simulink model "LGS_allFaultStuffDeleted"  (R2019b)
settings: Solver=FixedStepDiscrete  StartTime=0.0  StopTime=45.0  FixedStep=0.1  RelTol=1e-3
model workspace (MAT data in the model file):
  fipData : object (value not decoded)
  fipName : object (value not decoded)
  stepSize = 0.1
libraries: commrandsrc3 x16, simulink x3, LibFailureCondition x1
(part 4 of 7)

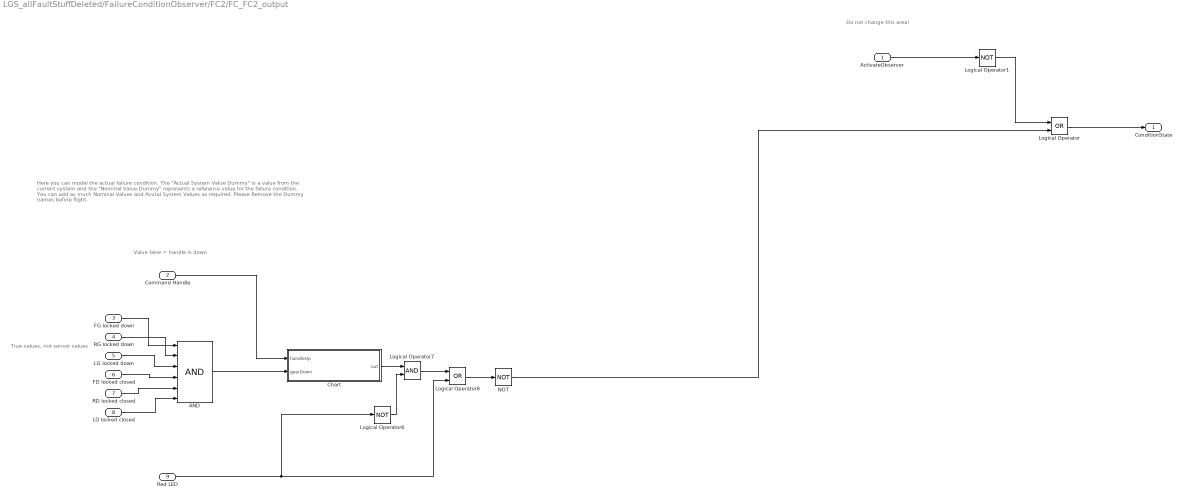
== system LGS_allFaultStuffDeleted/FailureConditionObserver/FC2/FC_FC2_output ==
  note: Here you can model the actual failure condition. The "Actual System Value Dummy" is a value from the current system and the "Nominal Value Dummy"
      | represents a reference value for the failure condition. You can add as much Nominal Values and Acutal System Values as required. Please Remove the
      | Dummy names before flight.
  note: Do not change this area!
  note: True values, not sensor values
  note: Value false = handle is down
  ActivateObserver : Inport
  Command Handle : Inport  Port=2
  FG locked down : Inport  Port=3
  RG locked down : Inport  Port=4
  LG locked down : Inport  Port=5
  FD locked closed : Inport  Port=6
  RD locked closed : Inport  Port=7
  LD locked closed : Inport  Port=8
  Red LED : Inport  Port=9
  AND : Logic  Inputs=6  IconShape=distinctive  AllPortsSameDT=off  OutDataTypeStr=boolean
  Chart : Stateflow chart  TreatAsAtomicUnit=on
  Logical Operator : Logic  Operator=OR  AllPortsSameDT=off  OutDataTypeStr=boolean
  Logical Operator1 : Logic  Operator=NOT  AllPortsSameDT=off  OutDataTypeStr=boolean
  Logical Operator6 : Logic  Operator=NOT  AllPortsSameDT=off  OutDataTypeStr=boolean
  Logical Operator7 : Logic  AllPortsSameDT=off  OutDataTypeStr=boolean
  Logical Operator8 : Logic  Operator=OR  AllPortsSameDT=off  OutDataTypeStr=boolean
  NOT : Logic  Operator=NOT  AllPortsSameDT=off  OutDataTypeStr=boolean
  ConditionState : Outport
  wires:
  ActivateObserver/1 -> Logical Operator1/1
  Logical Operator/1 -> ConditionState/1
  Logical Operator1/1 -> Logical Operator/1
  Logical Operator8/1 -> NOT/1
  Logical Operator7/1 -> Logical Operator8/1
  Logical Operator6/1 -> Logical Operator7/2
  Red LED/1 -> Logical Operator8/2, Logical Operator6/1
  LG locked down/1 -> AND/3
  RD locked closed/1 -> AND/5
  LD locked closed/1 -> AND/6
  FG locked down/1 -> AND/1
  Command Handle/1 -> Chart/1(handleUp)
  Chart/1(out) -> Logical Operator7/1
  RG locked down/1 -> AND/2
  FD locked closed/1 -> AND/4
  AND/1 -> Chart/2(gearDown)
  NOT/1 -> Logical Operator/2

== system LGS_allFaultStuffDeleted/FailureConditionObserver/FC3/ActualSystemCondition ==
  note: This section validates whether the failure condition to be observed will be evaluated. If the
      | last condition evaluates to false, the following conditions will not be evaluated!
      |
      | The last output should be evaluated to a boolean.
  Green LED : Inport
  Orange LED : Inport  Port=2
  Red LED : Inport  Port=3
  AND : Logic  Inputs=3  AllPortsSameDT=off  OutDataTypeStr=boolean
  NOT : Logic  Operator=NOT  AllPortsSameDT=off  OutDataTypeStr=boolean
  NOT1 : Logic  Operator=NOT  AllPortsSameDT=off  OutDataTypeStr=boolean
  "Activate Observer " : Outport
  wires:
  AND/1 -> "Activate Observer "/1
  NOT/1 -> AND/2
  Red LED/1 -> NOT1/1
  Orange LED/1 -> NOT/1
  Green LED/1 -> AND/1
  NOT1/1 -> AND/3

== system LGS_allFaultStuffDeleted/FailureConditionObserver/FC3/FC_FC3_output ==
  note: Here you can model the actual failure condition. The "Actual System Value Dummy" is a value from the current system and the "Nominal Value Dummy"
      | represents a reference value for the failure condition. You can add as much Nominal Values and Acutal System Values as required. Please Remove the
      | Dummy names before flight.
  note: Do not change this area!
  note: True values, not sensor values
  ActivateObserver : Inport
  FG locked down : Inport  Port=2
  RG locked down : Inport  Port=3
  LG locked down : Inport  Port=4
  FD locked closed1 : Inport  Port=5
  RD locked closed1 : Inport  Port=6
  LD locked closed1 : Inport  Port=7
  Logical Operator : Logic  AllPortsSameDT=off  OutDataTypeStr=boolean
  NAND : Logic  Operator=NAND  Inputs=6  IconShape=distinctive  AllPortsSameDT=off  OutDataTypeStr=boolean
  ConditionState : Outport
  wires:
  Logical Operator/1 -> ConditionState/1
  ActivateObserver/1 -> Logical Operator/1
  NAND/1 -> Logical Operator/2
  FG locked down/1 -> NAND/1
  FD locked closed1/1 -> NAND/4
  RD locked closed1/1 -> NAND/5
  RG locked down/1 -> NAND/2
  LG locked down/1 -> NAND/3
  LD locked closed1/1 -> NAND/6

== system LGS_allFaultStuffDeleted/Gears/FG shock absorber/sensor shock absorber ==
  note: [true, false]
  note: [true, false]
  note: [true, false]
  sensor input : Inport  OutDataTypeStr=boolean
  Bus Creator3 : BusCreator  Inputs=3
  FIP1 : Subsystem
  FIP2 : Subsystem
  FIP3 : Subsystem
  sensor output : Outport
  wires:
  FIP2/1(Out1) -> Bus Creator3/2  "signal2"
  FIP1/1(Out1) -> Bus Creator3/1  "signal1"
  FIP3/1(Out1) -> Bus Creator3/3  "signal3"
  sensor input/1 -> FIP3/1(In1), FIP2/1(In1), FIP1/1(In1)
  Bus Creator3/1 -> sensor output/1

== system LGS_allFaultStuffDeleted/Gears/LG shock absorber/sensor shock absorber ==
  note: [true, false]
  note: [true, false]
  sensor input : Inport  OutDataTypeStr=boolean
  Bus Creator3 : BusCreator  Inputs=3
  FIP1 : Subsystem
  FIP2 : Subsystem
  FIP3 : Subsystem
  sensor output : Outport
  wires:
  FIP2/1(Out1) -> Bus Creator3/2  "signal2"
  FIP1/1(Out1) -> Bus Creator3/1  "signal1"
  FIP3/1(Out1) -> Bus Creator3/3  "signal3"
  sensor input/1 -> FIP3/1(In1), FIP2/1(In1), FIP1/1(In1)
  Bus Creator3/1 -> sensor output/1

== system LGS_allFaultStuffDeleted/Gears/RG shock absorber/sensor shock absorber ==
  note: [true, false]
  sensor input : Inport  OutDataTypeStr=boolean
  Bus Creator3 : BusCreator  Inputs=3
  FIP1 : Subsystem
  FIP2 : Subsystem
  FIP3 : Subsystem
  sensor output : Outport
  wires:
  FIP2/1(Out1) -> Bus Creator3/2  "signal2"
  FIP1/1(Out1) -> Bus Creator3/1  "signal1"
  FIP3/1(Out1) -> Bus Creator3/3  "signal3"
  sensor input/1 -> FIP3/1(In1), FIP2/1(In1), FIP1/1(In1)
  Bus Creator3/1 -> sensor output/1

== system LGS_allFaultStuffDeleted/Gears/front gear cylinder/sensor locked extended ==
  note: [true, false]
  note: [true, false]
  note: [true, false]
  sensor input : Inport  OutDataTypeStr=boolean
  Bus Creator3 : BusCreator  Inputs=3
  FIP1 : Subsystem
  FIP2 : Subsystem
  FIP3 : Subsystem
  sensor output : Outport
  wires:
  FIP2/1(Out1) -> Bus Creator3/2  "signal2"
  FIP1/1(Out1) -> Bus Creator3/1  "signal1"
  FIP3/1(Out1) -> Bus Creator3/3  "signal3"
  sensor input/1 -> FIP3/1(In1), FIP2/1(In1), FIP1/1(In1)
  Bus Creator3/1 -> sensor output/1

== system LGS_allFaultStuffDeleted/Gears/front gear cylinder/sensor locked retracted ==
  note: [true, false]
  note: [true, false]
  note: [true, false]
  sensor input : Inport  OutDataTypeStr=boolean
  Bus Creator3 : BusCreator  Inputs=3
  FIP1 : Subsystem
  FIP2 : Subsystem
  FIP3 : Subsystem
  sensor output : Outport
  wires:
  FIP2/1(Out1) -> Bus Creator3/2  "signal2"
  FIP1/1(Out1) -> Bus Creator3/1  "signal1"
  FIP3/1(Out1) -> Bus Creator3/3  "signal3"
  sensor input/1 -> FIP3/1(In1), FIP2/1(In1), FIP1/1(In1)
  Bus Creator3/1 -> sensor output/1

== system LGS_allFaultStuffDeleted/Gears/left gear cylinder/sensor locked extended ==
  note: [true, false]
  note: [true, false]
  note: [true, false]
  sensor input : Inport  OutDataTypeStr=boolean
  Bus Creator3 : BusCreator  Inputs=3
  FIP1 : Subsystem
  FIP2 : Subsystem
  FIP3 : Subsystem
  sensor output : Outport
  wires:
  FIP2/1(Out1) -> Bus Creator3/2  "signal2"
  FIP1/1(Out1) -> Bus Creator3/1  "signal1"
  FIP3/1(Out1) -> Bus Creator3/3  "signal3"
  sensor input/1 -> FIP1/1(In1), FIP2/1(In1), FIP3/1(In1)
  Bus Creator3/1 -> sensor output/1

== system LGS_allFaultStuffDeleted/Gears/left gear cylinder/sensor locked retracted ==
  note: [true, false]
  note: [true, false]
  note: [true, false]
  sensor input : Inport  OutDataTypeStr=boolean
  Bus Creator3 : BusCreator  Inputs=3
  FIP1 : Subsystem
  FIP2 : Subsystem
  FIP3 : Subsystem
  sensor output : Outport
  wires:
  FIP2/1(Out1) -> Bus Creator3/2  "signal2"
  FIP1/1(Out1) -> Bus Creator3/1  "signal1"
  FIP3/1(Out1) -> Bus Creator3/3  "signal3"
  sensor input/1 -> FIP3/1(In1), FIP2/1(In1), FIP1/1(In1)
  Bus Creator3/1 -> sensor output/1

== system LGS_allFaultStuffDeleted/Gears/right gear cylinder/sensor locked extended ==
  note: [true, false]
  note: [true, false]
  note: [true, false]
  sensor input : Inport  OutDataTypeStr=boolean
  Bus Creator3 : BusCreator  Inputs=3
  FIP1 : Subsystem
  FIP2 : Subsystem
  FIP3 : Subsystem
  sensor output : Outport
  wires:
  FIP2/1(Out1) -> Bus Creator3/2  "signal2"
  FIP1/1(Out1) -> Bus Creator3/1  "signal1"
  FIP3/1(Out1) -> Bus Creator3/3  "signal3"
  sensor input/1 -> FIP2/1(In1), FIP3/1(In1), FIP1/1(In1)
  Bus Creator3/1 -> sensor output/1

== system LGS_allFaultStuffDeleted/Gears/right gear cylinder/sensor locked retracted ==
  note: [true, false]
  note: [true, false]
  note: [true, false]
  sensor input : Inport  OutDataTypeStr=boolean
  Bus Creator3 : BusCreator  Inputs=3
  FIP1 : Subsystem
  FIP2 : Subsystem
  FIP3 : Subsystem
  sensor output : Outport
  wires:
  FIP2/1(Out1) -> Bus Creator3/2  "signal2"
  FIP1/1(Out1) -> Bus Creator3/1  "signal1"
  FIP3/1(Out1) -> Bus Creator3/3  "signal3"
  sensor input/1 -> FIP3/1(In1), FIP2/1(In1), FIP1/1(In1)
  Bus Creator3/1 -> sensor output/1

== system LGS_allFaultStuffDeleted/Doors/front door zylinder/sensor locked closed/FIP1 ==
  In1 : Inport
  Out1 : Outport
  wires:
  In1/1 -> Out1/1

== system LGS_allFaultStuffDeleted/Doors/front door zylinder/sensor locked closed/FIP2 ==
  In1 : Inport
  Out1 : Outport
  wires:
  In1/1 -> Out1/1

== system LGS_allFaultStuffDeleted/Doors/front door zylinder/sensor locked closed/FIP3 ==
  In1 : Inport
  Out1 : Outport
  wires:
  In1/1 -> Out1/1

== system LGS_allFaultStuffDeleted/Doors/front door zylinder/sensor open/FIP1 ==
  In1 : Inport
  Out1 : Outport
  wires:
  In1/1 -> Out1/1

== system LGS_allFaultStuffDeleted/Doors/front door zylinder/sensor open/FIP2 ==
  In1 : Inport
  Out1 : Outport
  wires:
  In1/1 -> Out1/1

== system LGS_allFaultStuffDeleted/Doors/front door zylinder/sensor open/FIP3 ==
  In1 : Inport
  Out1 : Outport
  wires:
  In1/1 -> Out1/1

== system LGS_allFaultStuffDeleted/Doors/left door zylinder/sensor locked closed/FIP1 ==
  In1 : Inport
  Out1 : Outport
  wires:
  In1/1 -> Out1/1

== system LGS_allFaultStuffDeleted/Doors/left door zylinder/sensor locked closed/FIP2 ==
  In1 : Inport
  Out1 : Outport
  wires:
  In1/1 -> Out1/1

== system LGS_allFaultStuffDeleted/Doors/left door zylinder/sensor locked closed/FIP3 ==
  In1 : Inport
  Out1 : Outport
  wires:
  In1/1 -> Out1/1

== system LGS_allFaultStuffDeleted/Doors/left door zylinder/sensor open/FIP1 ==
  In1 : Inport
  Out1 : Outport
  wires:
  In1/1 -> Out1/1

== system LGS_allFaultStuffDeleted/Doors/left door zylinder/sensor open/FIP2 ==
  In1 : Inport
  Out1 : Outport
  wires:
  In1/1 -> Out1/1

== system LGS_allFaultStuffDeleted/Doors/left door zylinder/sensor open/FIP3 ==
  In1 : Inport
  Out1 : Outport
  wires:
  In1/1 -> Out1/1

== system LGS_allFaultStuffDeleted/Doors/right door zylinder/sensor locked closed/FIP1 ==
  In1 : Inport
  Out1 : Outport
  wires:
  In1/1 -> Out1/1

== system LGS_allFaultStuffDeleted/Doors/right door zylinder/sensor locked closed/FIP2 ==
  In1 : Inport
  Out1 : Outport
  wires:
  In1/1 -> Out1/1

== system LGS_allFaultStuffDeleted/Doors/right door zylinder/sensor locked closed/FIP3 ==
  In1 : Inport
  Out1 : Outport
  wires:
  In1/1 -> Out1/1

== system LGS_allFaultStuffDeleted/Doors/right door zylinder/sensor open/FIP1 ==
  In1 : Inport
  Out1 : Outport
  wires:
  In1/1 -> Out1/1

== system LGS_allFaultStuffDeleted/Doors/right door zylinder/sensor open/FIP2 ==
  In1 : Inport
  Out1 : Outport
  wires:
  In1/1 -> Out1/1

== system LGS_allFaultStuffDeleted/Doors/right door zylinder/sensor open/FIP3 ==
  In1 : Inport
  Out1 : Outport
  wires:
  In1/1 -> Out1/1

== system LGS_allFaultStuffDeleted/Gears/FG shock absorber/sensor shock absorber/FIP1 ==
  In1 : Inport
  Out1 : Outport
  wires:
  In1/1 -> Out1/1

== system LGS_allFaultStuffDeleted/Gears/FG shock absorber/sensor shock absorber/FIP2 ==
  In1 : Inport
  Out1 : Outport
  wires:
  In1/1 -> Out1/1

== system LGS_allFaultStuffDeleted/Gears/FG shock absorber/sensor shock absorber/FIP3 ==
  In1 : Inport
  Out1 : Outport
  wires:
  In1/1 -> Out1/1

== system LGS_allFaultStuffDeleted/Gears/LG shock absorber/sensor shock absorber/FIP1 ==
  In1 : Inport
  Out1 : Outport
  wires:
  In1/1 -> Out1/1

== system LGS_allFaultStuffDeleted/Gears/LG shock absorber/sensor shock absorber/FIP2 ==
  In1 : Inport
  Out1 : Outport
  wires:
  In1/1 -> Out1/1

== system LGS_allFaultStuffDeleted/Gears/LG shock absorber/sensor shock absorber/FIP3 ==
  In1 : Inport
  Out1 : Outport
  wires:
  In1/1 -> Out1/1

== system LGS_allFaultStuffDeleted/Gears/RG shock absorber/sensor shock absorber/FIP1 ==
  In1 : Inport
  Out1 : Outport
  wires:
  In1/1 -> Out1/1

== system LGS_allFaultStuffDeleted/Gears/RG shock absorber/sensor shock absorber/FIP2 ==
  In1 : Inport
  Out1 : Outport
  wires:
  In1/1 -> Out1/1

== system LGS_allFaultStuffDeleted/Gears/RG shock absorber/sensor shock absorber/FIP3 ==
  In1 : Inport
  Out1 : Outport
  wires:
  In1/1 -> Out1/1

== system LGS_allFaultStuffDeleted/Gears/front gear cylinder/sensor locked extended/FIP1 ==
  In1 : Inport
  Out1 : Outport
  wires:
  In1/1 -> Out1/1

== system LGS_allFaultStuffDeleted/Gears/front gear cylinder/sensor locked extended/FIP2 ==
  In1 : Inport
  Out1 : Outport
  wires:
  In1/1 -> Out1/1

== system LGS_allFaultStuffDeleted/Gears/front gear cylinder/sensor locked extended/FIP3 ==
  In1 : Inport
  Out1 : Outport
  wires:
  In1/1 -> Out1/1

== system LGS_allFaultStuffDeleted/Gears/front gear cylinder/sensor locked retracted/FIP1 ==
  In1 : Inport
  Out1 : Outport
  wires:
  In1/1 -> Out1/1

== system LGS_allFaultStuffDeleted/Gears/front gear cylinder/sensor locked retracted/FIP2 ==
  In1 : Inport
  Out1 : Outport
  wires:
  In1/1 -> Out1/1

== system LGS_allFaultStuffDeleted/Gears/front gear cylinder/sensor locked retracted/FIP3 ==
  In1 : Inport
  Out1 : Outport
  wires:
  In1/1 -> Out1/1

== system LGS_allFaultStuffDeleted/Gears/left gear cylinder/sensor locked extended/FIP1 ==
  In1 : Inport
  Out1 : Outport
  wires:
  In1/1 -> Out1/1

== system LGS_allFaultStuffDeleted/Gears/left gear cylinder/sensor locked extended/FIP2 ==
  In1 : Inport
  Out1 : Outport
  wires:
  In1/1 -> Out1/1

== system LGS_allFaultStuffDeleted/Gears/left gear cylinder/sensor locked extended/FIP3 ==
  In1 : Inport
  Out1 : Outport
  wires:
  In1/1 -> Out1/1

== system LGS_allFaultStuffDeleted/Gears/left gear cylinder/sensor locked retracted/FIP1 ==
  In1 : Inport
  Out1 : Outport
  wires:
  In1/1 -> Out1/1

== system LGS_allFaultStuffDeleted/Gears/left gear cylinder/sensor locked retracted/FIP2 ==
  In1 : Inport
  Out1 : Outport
  wires:
  In1/1 -> Out1/1

== system LGS_allFaultStuffDeleted/Gears/left gear cylinder/sensor locked retracted/FIP3 ==
  In1 : Inport
  Out1 : Outport
  wires:
  In1/1 -> Out1/1

== system LGS_allFaultStuffDeleted/Gears/right gear cylinder/sensor locked extended/FIP1 ==
  In1 : Inport
  Out1 : Outport
  wires:
  In1/1 -> Out1/1

== system LGS_allFaultStuffDeleted/Gears/right gear cylinder/sensor locked extended/FIP2 ==
  In1 : Inport
  Out1 : Outport
  wires:
  In1/1 -> Out1/1

== system LGS_allFaultStuffDeleted/Gears/right gear cylinder/sensor locked extended/FIP3 ==
  In1 : Inport
  Out1 : Outport
  wires:
  In1/1 -> Out1/1

== system LGS_allFaultStuffDeleted/Gears/right gear cylinder/sensor locked retracted/FIP1 ==
  In1 : Inport
  Out1 : Outport
  wires:
  In1/1 -> Out1/1

== system LGS_allFaultStuffDeleted/Gears/right gear cylinder/sensor locked retracted/FIP2 ==
  In1 : Inport
  Out1 : Outport
  wires:
  In1/1 -> Out1/1

== system LGS_allFaultStuffDeleted/Gears/right gear cylinder/sensor locked retracted/FIP3 ==
  In1 : Inport
  Out1 : Outport
  wires:
  In1/1 -> Out1/1

== stateflow chart LGS_allFaultStuffDeleted/Analogical switch and general electro-valve and pressure sensor/Analogical switch/analog Switch ==
  state state_analogSwitchOpenFail
    en: analogSwitchState = false;
  state state_analogSwitchOpen
    en: analogSwitchState = false;
    en: time = int8(1);
    du: time = time - 1;
  state state_analogSwitchOpened
    en: analogSwitchState = false;
  state state_analogSwitchClose
    en: analogSwitchState = false;
  state state_analogSwitchClosed
    en: analogSwitchState = true;
    en: time = int8(19);
    du: time = time - 1;
  state state_analogSwitchClosedFail
    en: analogSwitchState = true;
  state_analogSwitchOpen -> state_analogSwitchOpenFail [order 3] : [fail]
  (default) -> state_analogSwitchOpened
  state_analogSwitchOpen -> state_analogSwitchOpened [order 1] : [((time==0) && ~handleStateChanged) && ~fail]
  state_analogSwitchOpen -> state_analogSwitchClose [order 2] : [handleStateChanged && ~fail]
  state_analogSwitchOpened -> state_analogSwitchClose : [handleStateChanged && ~fail]
  state_analogSwitchClosed -> state_analogSwitchOpen [order 1] : [((time==0) && ~handleStateChanged) && ~fail]
  state_analogSwitchClose -> state_analogSwitchClosed
  state_analogSwitchClosed -> state_analogSwitchClosed [order 2] : [handleStateChanged && ~fail]
  state_analogSwitchClosed -> state_analogSwitchClosedFail [order 3] : [fail]
  data: handleStateChanged input boolean; analogSwitchState output boolean [0..1]; time local int8 [0..19]; fail input

== stateflow chart LGS_allFaultStuffDeleted/Digital Part/Computing module1/AnalogicalSwitchMonitoring ==
  state SwitchOpened
    entry: time = int8(21);
    during: time = time -1;
  note: If the analogical switch is seen closed 1.5 second after a time interval of 20
      | seconds during which the handle position has not changed, then the switch
      | is considered as invalid.
  state Idle
    entry: anomaly = false;
  state HandleMoved
  state CounterOrder
  note: If the analogical switch is seen open 1 second after the handle position has
      | changed, then the switch is considered as invalid.
  state Anomaly
    entry: anomaly = true;
  (default) -> Idle
  SwitchOpened -> Idle [order 2] : [((time == 0) && (~SwitchSignal))]
  HandleMoved -> SwitchOpened [order 2] : [((SwitchSignal) && (~HandleMoved))]
  SwitchOpened -> CounterOrder [order 3] : [(HandleMoved)]
  SwitchOpened -> Anomaly [order 1] : [((time == 0) && (SwitchSignal))]
  Idle -> HandleMoved : [(HandleMoved)]
  HandleMoved -> CounterOrder [order 3] : [(HandleMoved)]
  CounterOrder -> HandleMoved
  HandleMoved -> Anomaly [order 1] : [((~SwitchSignal) && (~HandleMoved))]
  data: HandleMoved input boolean; time local int8 [0..21]; SwitchSignal input boolean; anomaly output boolean

== stateflow chart LGS_allFaultStuffDeleted/Analogical switch and general electro-valve and pressure sensor/General EV/general EV ==
  state state_generalEVOpened
    en: generalEVPresure_out = false;
  state state_genralEVClose
    en: generalEVPresure_out = false;
  state state_generalEVClosed
    en: generalEVPresure_out = true;
  (default) -> state_generalEVOpened
  state_generalEVClosed -> state_generalEVOpened : [((~signal_in) || (~generalEVPresure_in)) && ~fail]
  state_generalEVOpened -> state_genralEVClose : [(signal_in && generalEVPresure_in && ~fail)]
  state_genralEVClose -> state_generalEVOpened [order 2] : [((~signal_in) || (~generalEVPresure_in)) && ~fail]
  state_genralEVClose -> state_generalEVClosed [order 1] : [(signal_in && generalEVPresure_in && ~fail)]
  data: generalEVPresure_in input boolean; signal_in input boolean; generalEVPresure_out output boolean [0..1]; fail input

== stateflow chart LGS_allFaultStuffDeleted/Digital Part/Computing module1/DoorMotionMonitoring ==
  state Idle
    entry: anomaly = false;
  state CloseDoors
    entry: time = int8(6);
    during: time = time -1;
  note: if the control software does not see the value door closed[x] = true for all
      | x ∈ {front, left, right} 7 seconds after stimulation of the closure electro-valve,
      | then the doors are considered as blocked and an anomaly is detected.
  state Succeeded
  state OpenDoors
    entry: time = int8(6);
    during: time = time - 1;
  note: if the control software does not see the value door open[x] = false for all x ∈ {front, left, right} 7 seconds after stimulation of the closure electro-valve, then the doors are considered as blocked and an anomaly is detected.
  state CounterOrder
  note: if the control software does not see the value door open[x] = true for all
      | x ∈ {front, left, right} 7 seconds after stimulation of the opening electrovalve,
      | then the doors are considered as blocked and an anomaly is detected.
  state DoorsBlocked
    entry: anomaly = true;
  note: if the control software does not see the value door closed[x] = false for all
      | x ∈ {front, left, right} 7 seconds after stimulation of the opening electro-valve,
      | then the doors are considered as blocked and an anomaly is detected.
  (default) -> Idle
  CloseDoors -> DoorsBlocked [order 2] : [((time == 0) && (~AllDoorsClosed))]
  Idle -> CloseDoors [order 2] : [((CloseDoorValve) && (~AllDoorsClosed))]
  CloseDoors -> DoorsBlocked [order 3] : [((time == 0) && (AllDoorsOpen))]
  Succeeded -> Idle
  CloseDoors -> Succeeded [order 1] : [(((time == 0) && (AllDoorsClosed)) && (~AllDoorsOpen))]
  CounterOrder -> CloseDoors [order 2] : [(CloseDoorValve)]
  CloseDoors -> CounterOrder [order 4] : [(~CloseDoorValve)]
  Idle -> OpenDoors [order 1] : [((OpenDoorValve) && (~AllDoorsOpen))]
  OpenDoors -> Succeeded [order 2] : [(((time == 0) && (~AllDoorsClosed)) && (AllDoorsOpen))]
  CounterOrder -> OpenDoors [order 1] : [(OpenDoorValve)]
  OpenDoors -> CounterOrder [order 4] : [(~OpenDoorValve)]
  OpenDoors -> DoorsBlocked [order 1] : [((time == 0) && (AllDoorsClosed))]
  OpenDoors -> DoorsBlocked [order 3] : [((time == 0) && (~AllDoorsOpen))]
  data: OpenDoorValve input boolean; time local int8 [0..6]; CloseDoorValve input boolean; anomaly output boolean; AllDoorsClosed input boolean; AllDoorsOpen input boolean

== stateflow chart LGS_allFaultStuffDeleted/Digital Part/Computing module1/GearMotionMonitoring ==
  state ContinueExtending
    entry: time = int8(2);
    during: time = time -1;
  note: if the control software does not see the value gear extended[x] = true for all x ∈ {front, left, right} 10 seconds after stimulation of the extension electrovalve, then the gears are considered as blocked and an anomaly is detected.
  state Idle
    entry: anomaly = false;
  state ExtendGears
    entry: time = int8(6);
    during: time = time -1;
  state RetractGears
    entry: time = int8(6);
    during: time = time - 1;
  state ContinueRetracting
    entry: time = int8(2);
    during: time = time -1;
  state Succeeded
  note: if the control software does not see the value gear retracted[x] = false for all x ∈ {front, left, right} 7 seconds after stimulation of the extension electrovalve, then the gears are considered as blocked and an anomaly is detected.
  state GearsBlocked
    entry: anomaly = true;
  state CounterOrder
  note: if the control software does not see the value gear retracted[x] = true for all x ∈ {front, left, right} 10 seconds after stimulation of the retraction electrovalve, then the gears are considered as blocked and an anomaly is detected.
  note: if the control software does not see the value gear extended[x] = false for all
      | x ∈ {front, left, right} 7 seconds after stimulation of the retraction electrovalve,
      | then the gears are considered as blocked and an anomaly is detected.
  (default) -> Idle
  ExtendGears -> ContinueExtending [order 1] : [((time == 0) && (~AllGearsRetracted))]
  Idle -> ExtendGears [order 2] : [(ExtensionValve)]
  ExtendGears -> GearsBlocked [order 2] : [((time == 0) && (AllGearsRetracted))]
  Succeeded -> Idle
  ExtendGears -> CounterOrder [order 3] : [(~ExtensionValve)]
  ContinueExtending -> GearsBlocked [order 2] : [((time == 0) && (~AllGearsExtended))]
  CounterOrder -> ExtendGears [order 2] : [(ExtensionValve)]
  Idle -> RetractGears [order 1] : [(RetractionValve)]
  ContinueExtending -> CounterOrder [order 3] : [(~ExtensionValve)]
  ContinueExtending -> Succeeded [order 1] : [((time == 0) && (AllGearsExtended))]
  RetractGears -> ContinueRetracting [order 2] : [((time == 0) && (~AllGearsExtended))]
  ContinueRetracting -> Succeeded [order 1] : [((time == 0) && (AllGearsRetracted))]
  CounterOrder -> RetractGears [order 1] : [(RetractionValve)]
  ContinueRetracting -> GearsBlocked [order 2] : [((time == 0) && (~AllGearsRetracted))]
  RetractGears -> GearsBlocked [order 1] : [((time == 0) && (AllGearsExtended))]
  RetractGears -> CounterOrder [order 3] : [(~RetractionValve)]
  ContinueRetracting -> CounterOrder [order 3] : [(~RetractionValve)]
  data: time local int8 [0..6]; anomaly output boolean; AllGearsExtended input boolean; AllGearsRetracted input boolean; ExtensionValve input boolean; RetractionValve input boolean

== stateflow chart LGS_allFaultStuffDeleted/Digital Part/Computing module1/GenericMonitoring/GenericMonitoring2 ==
  state SensorValid
    entry: anomaly = false;
  state Channel1Invalid
  state SensorInvalid
    entry: anomaly = true;
  note: If at t the three channels are considered as valid and are equal, then the
      | value considered by the control software is this common value.
  state Channel2Invalid
  note: If a channel has been eliminated previously, and if at t the two remaining
      | channels are not equal, then the sensor is definitely considered as invalid.
  state Channel3Invalid
  note: If at t one channel is different from the two others for the first time (i.e.,
      | the three channels were considered as valid up to t), then this channel is
      | considered as invalid and is definitely eliminated. Only the two remaining
      | channels are considered in the future. At time t, the value considered by the
      | control software is the common value of the two remaining channels.
  (default) -> SensorValid
  SensorValid -> Channel1Invalid [order 1] : [(((Channel3&&Channel2) || ((~Channel3)&&(~Channel2))) && ((Channel1 && (~Channel2)) || ((~Channel1) && Channel2)))]
  Channel1Invalid -> SensorInvalid : [((Channel2 && (~Channel3)) || ((~Channel2) && Channel3))]
  SensorValid -> Channel2Invalid [order 2] : [(((Channel1&&Channel3) || ((~Channel1)&&(~Channel3))) && ((Channel1 && (~Channel2)) || ((~Channel1) && Channel2)))]
  SensorValid -> Channel3Invalid [order 3] : [(((Channel1&&Channel2) || ((~Channel1)&&(~Channel2))) && ((Channel1 && (~Channel3)) || ((~Channel1) && Channel3)))]
  Channel2Invalid -> SensorInvalid : [((Channel1 && (~Channel3)) || ((~Channel1) && Channel3))]
  Channel3Invalid -> SensorInvalid : [((Channel2 && (~Channel1)) || ((~Channel2) && Channel1))]
  data: Channel1 input boolean; Channel2 input boolean; Channel3 input boolean; anomaly output boolean

== stateflow chart LGS_allFaultStuffDeleted/Digital Part/Computing module1/GenericMonitoring1/GenericMonitoring2 ==
  state SensorValid
    entry: anomaly = false;
  state Channel1Invalid
  state SensorInvalid
    entry: anomaly = true;
  note: If at t the three channels are considered as valid and are equal, then the
      | value considered by the control software is this common value.
  state Channel2Invalid
  note: If a channel has been eliminated previously, and if at t the two remaining
      | channels are not equal, then the sensor is definitely considered as invalid.
  state Channel3Invalid
  note: If at t one channel is different from the two others for the first time (i.e.,
      | the three channels were considered as valid up to t), then this channel is
      | considered as invalid and is definitely eliminated. Only the two remaining
      | channels are considered in the future. At time t, the value considered by the
      | control software is the common value of the two remaining channels.
  (default) -> SensorValid
  SensorValid -> Channel1Invalid [order 1] : [(((Channel3&&Channel2) || ((~Channel3)&&(~Channel2))) && ((Channel1 && (~Channel2)) || ((~Channel1) && Channel2)))]
  Channel1Invalid -> SensorInvalid : [((Channel2 && (~Channel3)) || ((~Channel2) && Channel3))]
  SensorValid -> Channel2Invalid [order 2] : [(((Channel1&&Channel3) || ((~Channel1)&&(~Channel3))) && ((Channel1 && (~Channel2)) || ((~Channel1) && Channel2)))]
  SensorValid -> Channel3Invalid [order 3] : [(((Channel1&&Channel2) || ((~Channel1)&&(~Channel2))) && ((Channel1 && (~Channel3)) || ((~Channel1) && Channel3)))]
  Channel2Invalid -> SensorInvalid : [((Channel1 && (~Channel3)) || ((~Channel1) && Channel3))]
  Channel3Invalid -> SensorInvalid : [((Channel2 && (~Channel1)) || ((~Channel2) && Channel1))]
  data: Channel1 input boolean; Channel2 input boolean; Channel3 input boolean; anomaly output boolean

== stateflow chart LGS_allFaultStuffDeleted/Digital Part/Computing module1/GenericMonitoring10/GenericMonitoring2 ==
  state SensorValid
    entry: anomaly = false;
  state Channel1Invalid
  state SensorInvalid
    entry: anomaly = true;
  note: If at t the three channels are considered as valid and are equal, then the
      | value considered by the control software is this common value.
  state Channel2Invalid
  note: If a channel has been eliminated previously, and if at t the two remaining
      | channels are not equal, then the sensor is definitely considered as invalid.
  state Channel3Invalid
  note: If at t one channel is different from the two others for the first time (i.e.,
      | the three channels were considered as valid up to t), then this channel is
      | considered as invalid and is definitely eliminated. Only the two remaining
      | channels are considered in the future. At time t, the value considered by the
      | control software is the common value of the two remaining channels.
  (default) -> SensorValid
  SensorValid -> Channel1Invalid [order 1] : [(((Channel3&&Channel2) || ((~Channel3)&&(~Channel2))) && ((Channel1 && (~Channel2)) || ((~Channel1) && Channel2)))]
  Channel1Invalid -> SensorInvalid : [((Channel2 && (~Channel3)) || ((~Channel2) && Channel3))]
  SensorValid -> Channel2Invalid [order 2] : [(((Channel1&&Channel3) || ((~Channel1)&&(~Channel3))) && ((Channel1 && (~Channel2)) || ((~Channel1) && Channel2)))]
  SensorValid -> Channel3Invalid [order 3] : [(((Channel1&&Channel2) || ((~Channel1)&&(~Channel2))) && ((Channel1 && (~Channel3)) || ((~Channel1) && Channel3)))]
  Channel2Invalid -> SensorInvalid : [((Channel1 && (~Channel3)) || ((~Channel1) && Channel3))]
  Channel3Invalid -> SensorInvalid : [((Channel2 && (~Channel1)) || ((~Channel2) && Channel1))]
  data: Channel1 input boolean; Channel2 input boolean; Channel3 input boolean; anomaly output boolean

== stateflow chart LGS_allFaultStuffDeleted/Digital Part/Computing module1/GenericMonitoring11/GenericMonitoring2 ==
  state SensorValid
    entry: anomaly = false;
  state Channel1Invalid
  state SensorInvalid
    entry: anomaly = true;
  note: If at t the three channels are considered as valid and are equal, then the
      | value considered by the control software is this common value.
  state Channel2Invalid
  note: If a channel has been eliminated previously, and if at t the two remaining
      | channels are not equal, then the sensor is definitely considered as invalid.
  state Channel3Invalid
  note: If at t one channel is different from the two others for the first time (i.e.,
      | the three channels were considered as valid up to t), then this channel is
      | considered as invalid and is definitely eliminated. Only the two remaining
      | channels are considered in the future. At time t, the value considered by the
      | control software is the common value of the two remaining channels.
  (default) -> SensorValid
  SensorValid -> Channel1Invalid [order 1] : [(((Channel3&&Channel2) || ((~Channel3)&&(~Channel2))) && ((Channel1 && (~Channel2)) || ((~Channel1) && Channel2)))]
  Channel1Invalid -> SensorInvalid : [((Channel2 && (~Channel3)) || ((~Channel2) && Channel3))]
  SensorValid -> Channel2Invalid [order 2] : [(((Channel1&&Channel3) || ((~Channel1)&&(~Channel3))) && ((Channel1 && (~Channel2)) || ((~Channel1) && Channel2)))]
  SensorValid -> Channel3Invalid [order 3] : [(((Channel1&&Channel2) || ((~Channel1)&&(~Channel2))) && ((Channel1 && (~Channel3)) || ((~Channel1) && Channel3)))]
  Channel2Invalid -> SensorInvalid : [((Channel1 && (~Channel3)) || ((~Channel1) && Channel3))]
  Channel3Invalid -> SensorInvalid : [((Channel2 && (~Channel1)) || ((~Channel2) && Channel1))]
  data: Channel1 input boolean; Channel2 input boolean; Channel3 input boolean; anomaly output boolean

== stateflow chart LGS_allFaultStuffDeleted/Digital Part/Computing module1/GenericMonitoring12/GenericMonitoring2 ==
  state SensorValid
    entry: anomaly = false;
  state Channel1Invalid
  state SensorInvalid
    entry: anomaly = true;
  note: If at t the three channels are considered as valid and are equal, then the
      | value considered by the control software is this common value.
  state Channel2Invalid
  note: If a channel has been eliminated previously, and if at t the two remaining
      | channels are not equal, then the sensor is definitely considered as invalid.
  state Channel3Invalid
  note: If at t one channel is different from the two others for the first time (i.e.,
      | the three channels were considered as valid up to t), then this channel is
      | considered as invalid and is definitely eliminated. Only the two remaining
      | channels are considered in the future. At time t, the value considered by the
      | control software is the common value of the two remaining channels.
  (default) -> SensorValid
  SensorValid -> Channel1Invalid [order 1] : [(((Channel3&&Channel2) || ((~Channel3)&&(~Channel2))) && ((Channel1 && (~Channel2)) || ((~Channel1) && Channel2)))]
  Channel1Invalid -> SensorInvalid : [((Channel2 && (~Channel3)) || ((~Channel2) && Channel3))]
  SensorValid -> Channel2Invalid [order 2] : [(((Channel1&&Channel3) || ((~Channel1)&&(~Channel3))) && ((Channel1 && (~Channel2)) || ((~Channel1) && Channel2)))]
  SensorValid -> Channel3Invalid [order 3] : [(((Channel1&&Channel2) || ((~Channel1)&&(~Channel2))) && ((Channel1 && (~Channel3)) || ((~Channel1) && Channel3)))]
  Channel2Invalid -> SensorInvalid : [((Channel1 && (~Channel3)) || ((~Channel1) && Channel3))]
  Channel3Invalid -> SensorInvalid : [((Channel2 && (~Channel1)) || ((~Channel2) && Channel1))]
  data: Channel1 input boolean; Channel2 input boolean; Channel3 input boolean; anomaly output boolean

== stateflow chart LGS_allFaultStuffDeleted/Digital Part/Computing module1/GenericMonitoring13/GenericMonitoring2 ==
  state SensorValid
    entry: anomaly = false;
  state Channel1Invalid
  state SensorInvalid
    entry: anomaly = true;
  note: If at t the three channels are considered as valid and are equal, then the
      | value considered by the control software is this common value.
  state Channel2Invalid
  note: If a channel has been eliminated previously, and if at t the two remaining
      | channels are not equal, then the sensor is definitely considered as invalid.
  state Channel3Invalid
  note: If at t one channel is different from the two others for the first time (i.e.,
      | the three channels were considered as valid up to t), then this channel is
      | considered as invalid and is definitely eliminated. Only the two remaining
      | channels are considered in the future. At time t, the value considered by the
      | control software is the common value of the two remaining channels.
  (default) -> SensorValid
  SensorValid -> Channel1Invalid [order 1] : [(((Channel3&&Channel2) || ((~Channel3)&&(~Channel2))) && ((Channel1 && (~Channel2)) || ((~Channel1) && Channel2)))]
  Channel1Invalid -> SensorInvalid : [((Channel2 && (~Channel3)) || ((~Channel2) && Channel3))]
  SensorValid -> Channel2Invalid [order 2] : [(((Channel1&&Channel3) || ((~Channel1)&&(~Channel3))) && ((Channel1 && (~Channel2)) || ((~Channel1) && Channel2)))]
  SensorValid -> Channel3Invalid [order 3] : [(((Channel1&&Channel2) || ((~Channel1)&&(~Channel2))) && ((Channel1 && (~Channel3)) || ((~Channel1) && Channel3)))]
  Channel2Invalid -> SensorInvalid : [((Channel1 && (~Channel3)) || ((~Channel1) && Channel3))]
  Channel3Invalid -> SensorInvalid : [((Channel2 && (~Channel1)) || ((~Channel2) && Channel1))]
  data: Channel1 input boolean; Channel2 input boolean; Channel3 input boolean; anomaly output boolean

== stateflow chart LGS_allFaultStuffDeleted/Digital Part/Computing module1/GenericMonitoring14/GenericMonitoring2 ==
  state SensorValid
    entry: anomaly = false;
  state Channel1Invalid
  state SensorInvalid
    entry: anomaly = true;
  note: If at t the three channels are considered as valid and are equal, then the
      | value considered by the control software is this common value.
  state Channel2Invalid
  note: If a channel has been eliminated previously, and if at t the two remaining
      | channels are not equal, then the sensor is definitely considered as invalid.
  state Channel3Invalid
  note: If at t one channel is different from the two others for the first time (i.e.,
      | the three channels were considered as valid up to t), then this channel is
      | considered as invalid and is definitely eliminated. Only the two remaining
      | channels are considered in the future. At time t, the value considered by the
      | control software is the common value of the two remaining channels.
  (default) -> SensorValid
  SensorValid -> Channel1Invalid [order 1] : [(((Channel3&&Channel2) || ((~Channel3)&&(~Channel2))) && ((Channel1 && (~Channel2)) || ((~Channel1) && Channel2)))]
  Channel1Invalid -> SensorInvalid : [((Channel2 && (~Channel3)) || ((~Channel2) && Channel3))]
  SensorValid -> Channel2Invalid [order 2] : [(((Channel1&&Channel3) || ((~Channel1)&&(~Channel3))) && ((Channel1 && (~Channel2)) || ((~Channel1) && Channel2)))]
  SensorValid -> Channel3Invalid [order 3] : [(((Channel1&&Channel2) || ((~Channel1)&&(~Channel2))) && ((Channel1 && (~Channel3)) || ((~Channel1) && Channel3)))]
  Channel2Invalid -> SensorInvalid : [((Channel1 && (~Channel3)) || ((~Channel1) && Channel3))]
  Channel3Invalid -> SensorInvalid : [((Channel2 && (~Channel1)) || ((~Channel2) && Channel1))]
  data: Channel1 input boolean; Channel2 input boolean; Channel3 input boolean; anomaly output boolean

== stateflow chart LGS_allFaultStuffDeleted/Digital Part/Computing module1/GenericMonitoring2/GenericMonitoring2 ==
  state SensorValid
    entry: anomaly = false;
  state Channel1Invalid
  state SensorInvalid
    entry: anomaly = true;
  note: If at t the three channels are considered as valid and are equal, then the
      | value considered by the control software is this common value.
  state Channel2Invalid
  note: If a channel has been eliminated previously, and if at t the two remaining
      | channels are not equal, then the sensor is definitely considered as invalid.
  state Channel3Invalid
  note: If at t one channel is different from the two others for the first time (i.e.,
      | the three channels were considered as valid up to t), then this channel is
      | considered as invalid and is definitely eliminated. Only the two remaining
      | channels are considered in the future. At time t, the value considered by the
      | control software is the common value of the two remaining channels.
  (default) -> SensorValid
  SensorValid -> Channel1Invalid [order 1] : [(((Channel3&&Channel2) || ((~Channel3)&&(~Channel2))) && ((Channel1 && (~Channel2)) || ((~Channel1) && Channel2)))]
  Channel1Invalid -> SensorInvalid : [((Channel2 && (~Channel3)) || ((~Channel2) && Channel3))]
  SensorValid -> Channel2Invalid [order 2] : [(((Channel1&&Channel3) || ((~Channel1)&&(~Channel3))) && ((Channel1 && (~Channel2)) || ((~Channel1) && Channel2)))]
  SensorValid -> Channel3Invalid [order 3] : [(((Channel1&&Channel2) || ((~Channel1)&&(~Channel2))) && ((Channel1 && (~Channel3)) || ((~Channel1) && Channel3)))]
  Channel2Invalid -> SensorInvalid : [((Channel1 && (~Channel3)) || ((~Channel1) && Channel3))]
  Channel3Invalid -> SensorInvalid : [((Channel2 && (~Channel1)) || ((~Channel2) && Channel1))]
  data: Channel1 input boolean; Channel2 input boolean; Channel3 input boolean; anomaly output boolean

== stateflow chart LGS_allFaultStuffDeleted/Digital Part/Computing module1/GenericMonitoring3/GenericMonitoring2 ==
  state SensorValid
    entry: anomaly = false;
  state Channel1Invalid
  state SensorInvalid
    entry: anomaly = true;
  note: If at t the three channels are considered as valid and are equal, then the
      | value considered by the control software is this common value.
  state Channel2Invalid
  note: If a channel has been eliminated previously, and if at t the two remaining
      | channels are not equal, then the sensor is definitely considered as invalid.
  state Channel3Invalid
  note: If at t one channel is different from the two others for the first time (i.e.,
      | the three channels were considered as valid up to t), then this channel is
      | considered as invalid and is definitely eliminated. Only the two remaining
      | channels are considered in the future. At time t, the value considered by the
      | control software is the common value of the two remaining channels.
  (default) -> SensorValid
  SensorValid -> Channel1Invalid [order 1] : [(((Channel3&&Channel2) || ((~Channel3)&&(~Channel2))) && ((Channel1 && (~Channel2)) || ((~Channel1) && Channel2)))]
  Channel1Invalid -> SensorInvalid : [((Channel2 && (~Channel3)) || ((~Channel2) && Channel3))]
  SensorValid -> Channel2Invalid [order 2] : [(((Channel1&&Channel3) || ((~Channel1)&&(~Channel3))) && ((Channel1 && (~Channel2)) || ((~Channel1) && Channel2)))]
  SensorValid -> Channel3Invalid [order 3] : [(((Channel1&&Channel2) || ((~Channel1)&&(~Channel2))) && ((Channel1 && (~Channel3)) || ((~Channel1) && Channel3)))]
  Channel2Invalid -> SensorInvalid : [((Channel1 && (~Channel3)) || ((~Channel1) && Channel3))]
  Channel3Invalid -> SensorInvalid : [((Channel2 && (~Channel1)) || ((~Channel2) && Channel1))]
  data: Channel1 input boolean; Channel2 input boolean; Channel3 input boolean; anomaly output boolean

== stateflow chart LGS_allFaultStuffDeleted/Digital Part/Computing module1/GenericMonitoring4/GenericMonitoring2 ==
  state SensorValid
    entry: anomaly = false;
  state Channel1Invalid
  state SensorInvalid
    entry: anomaly = true;
  note: If at t the three channels are considered as valid and are equal, then the
      | value considered by the control software is this common value.
  state Channel2Invalid
  note: If a channel has been eliminated previously, and if at t the two remaining
      | channels are not equal, then the sensor is definitely considered as invalid.
  state Channel3Invalid
  note: If at t one channel is different from the two others for the first time (i.e.,
      | the three channels were considered as valid up to t), then this channel is
      | considered as invalid and is definitely eliminated. Only the two remaining
      | channels are considered in the future. At time t, the value considered by the
      | control software is the common value of the two remaining channels.
  (default) -> SensorValid
  SensorValid -> Channel1Invalid [order 1] : [(((Channel3&&Channel2) || ((~Channel3)&&(~Channel2))) && ((Channel1 && (~Channel2)) || ((~Channel1) && Channel2)))]
  Channel1Invalid -> SensorInvalid : [((Channel2 && (~Channel3)) || ((~Channel2) && Channel3))]
  SensorValid -> Channel2Invalid [order 2] : [(((Channel1&&Channel3) || ((~Channel1)&&(~Channel3))) && ((Channel1 && (~Channel2)) || ((~Channel1) && Channel2)))]
  SensorValid -> Channel3Invalid [order 3] : [(((Channel1&&Channel2) || ((~Channel1)&&(~Channel2))) && ((Channel1 && (~Channel3)) || ((~Channel1) && Channel3)))]
  Channel2Invalid -> SensorInvalid : [((Channel1 && (~Channel3)) || ((~Channel1) && Channel3))]
  Channel3Invalid -> SensorInvalid : [((Channel2 && (~Channel1)) || ((~Channel2) && Channel1))]
  data: Channel1 input boolean; Channel2 input boolean; Channel3 input boolean; anomaly output boolean

== stateflow chart LGS_allFaultStuffDeleted/Digital Part/Computing module1/GenericMonitoring5/GenericMonitoring2 ==
  state SensorValid
    entry: anomaly = false;
  state Channel1Invalid
  state SensorInvalid
    entry: anomaly = true;
  note: If at t the three channels are considered as valid and are equal, then the
      | value considered by the control software is this common value.
  state Channel2Invalid
  note: If a channel has been eliminated previously, and if at t the two remaining
      | channels are not equal, then the sensor is definitely considered as invalid.
  state Channel3Invalid
  note: If at t one channel is different from the two others for the first time (i.e.,
      | the three channels were considered as valid up to t), then this channel is
      | considered as invalid and is definitely eliminated. Only the two remaining
      | channels are considered in the future. At time t, the value considered by the
      | control software is the common value of the two remaining channels.
  (default) -> SensorValid
  SensorValid -> Channel1Invalid [order 1] : [(((Channel3&&Channel2) || ((~Channel3)&&(~Channel2))) && ((Channel1 && (~Channel2)) || ((~Channel1) && Channel2)))]
  Channel1Invalid -> SensorInvalid : [((Channel2 && (~Channel3)) || ((~Channel2) && Channel3))]
  SensorValid -> Channel2Invalid [order 2] : [(((Channel1&&Channel3) || ((~Channel1)&&(~Channel3))) && ((Channel1 && (~Channel2)) || ((~Channel1) && Channel2)))]
  SensorValid -> Channel3Invalid [order 3] : [(((Channel1&&Channel2) || ((~Channel1)&&(~Channel2))) && ((Channel1 && (~Channel3)) || ((~Channel1) && Channel3)))]
  Channel2Invalid -> SensorInvalid : [((Channel1 && (~Channel3)) || ((~Channel1) && Channel3))]
  Channel3Invalid -> SensorInvalid : [((Channel2 && (~Channel1)) || ((~Channel2) && Channel1))]
  data: Channel1 input boolean; Channel2 input boolean; Channel3 input boolean; anomaly output boolean

== stateflow chart LGS_allFaultStuffDeleted/Digital Part/Computing module1/GenericMonitoring6/GenericMonitoring2 ==
  state SensorValid
    entry: anomaly = false;
  state Channel1Invalid
  state SensorInvalid
    entry: anomaly = true;
  note: If at t the three channels are considered as valid and are equal, then the
      | value considered by the control software is this common value.
  state Channel2Invalid
  note: If a channel has been eliminated previously, and if at t the two remaining
      | channels are not equal, then the sensor is definitely considered as invalid.
  state Channel3Invalid
  note: If at t one channel is different from the two others for the first time (i.e.,
      | the three channels were considered as valid up to t), then this channel is
      | considered as invalid and is definitely eliminated. Only the two remaining
      | channels are considered in the future. At time t, the value considered by the
      | control software is the common value of the two remaining channels.
  (default) -> SensorValid
  SensorValid -> Channel1Invalid [order 1] : [(((Channel3&&Channel2) || ((~Channel3)&&(~Channel2))) && ((Channel1 && (~Channel2)) || ((~Channel1) && Channel2)))]
  Channel1Invalid -> SensorInvalid : [((Channel2 && (~Channel3)) || ((~Channel2) && Channel3))]
  SensorValid -> Channel2Invalid [order 2] : [(((Channel1&&Channel3) || ((~Channel1)&&(~Channel3))) && ((Channel1 && (~Channel2)) || ((~Channel1) && Channel2)))]
  SensorValid -> Channel3Invalid [order 3] : [(((Channel1&&Channel2) || ((~Channel1)&&(~Channel2))) && ((Channel1 && (~Channel3)) || ((~Channel1) && Channel3)))]
  Channel2Invalid -> SensorInvalid : [((Channel1 && (~Channel3)) || ((~Channel1) && Channel3))]
  Channel3Invalid -> SensorInvalid : [((Channel2 && (~Channel1)) || ((~Channel2) && Channel1))]
  data: Channel1 input boolean; Channel2 input boolean; Channel3 input boolean; anomaly output boolean

== stateflow chart LGS_allFaultStuffDeleted/Digital Part/Computing module1/GenericMonitoring7/GenericMonitoring2 ==
  state SensorValid
    entry: anomaly = false;
  state Channel1Invalid
  state SensorInvalid
    entry: anomaly = true;
  note: If at t the three channels are considered as valid and are equal, then the
      | value considered by the control software is this common value.
  state Channel2Invalid
  note: If a channel has been eliminated previously, and if at t the two remaining
      | channels are not equal, then the sensor is definitely considered as invalid.
  state Channel3Invalid
  note: If at t one channel is different from the two others for the first time (i.e.,
      | the three channels were considered as valid up to t), then this channel is
      | considered as invalid and is definitely eliminated. Only the two remaining
      | channels are considered in the future. At time t, the value considered by the
      | control software is the common value of the two remaining channels.
  (default) -> SensorValid
  SensorValid -> Channel1Invalid [order 1] : [(((Channel3&&Channel2) || ((~Channel3)&&(~Channel2))) && ((Channel1 && (~Channel2)) || ((~Channel1) && Channel2)))]
  Channel1Invalid -> SensorInvalid : [((Channel2 && (~Channel3)) || ((~Channel2) && Channel3))]
  SensorValid -> Channel2Invalid [order 2] : [(((Channel1&&Channel3) || ((~Channel1)&&(~Channel3))) && ((Channel1 && (~Channel2)) || ((~Channel1) && Channel2)))]
  SensorValid -> Channel3Invalid [order 3] : [(((Channel1&&Channel2) || ((~Channel1)&&(~Channel2))) && ((Channel1 && (~Channel3)) || ((~Channel1) && Channel3)))]
  Channel2Invalid -> SensorInvalid : [((Channel1 && (~Channel3)) || ((~Channel1) && Channel3))]
  Channel3Invalid -> SensorInvalid : [((Channel2 && (~Channel1)) || ((~Channel2) && Channel1))]
  data: Channel1 input boolean; Channel2 input boolean; Channel3 input boolean; anomaly output boolean
